simulink model "AutonomousDriving"  (R2018a)
settings: Solver=FixedStepAuto  StartTime=0.0  StopTime=inf  FixedStep=0.1  RelTol=1e-3
PreLoadFcn:
  | load('init.mat')
undefined symbols (not defined in the file): DiscIntNeverNeededParam, gray, init, Rec, SDTV
libraries: vrlib x7, simulink x3, PiCar_library x2, visionconversions x1
settings Model: Creator=al.hermann  LastModifiedBy=Tim

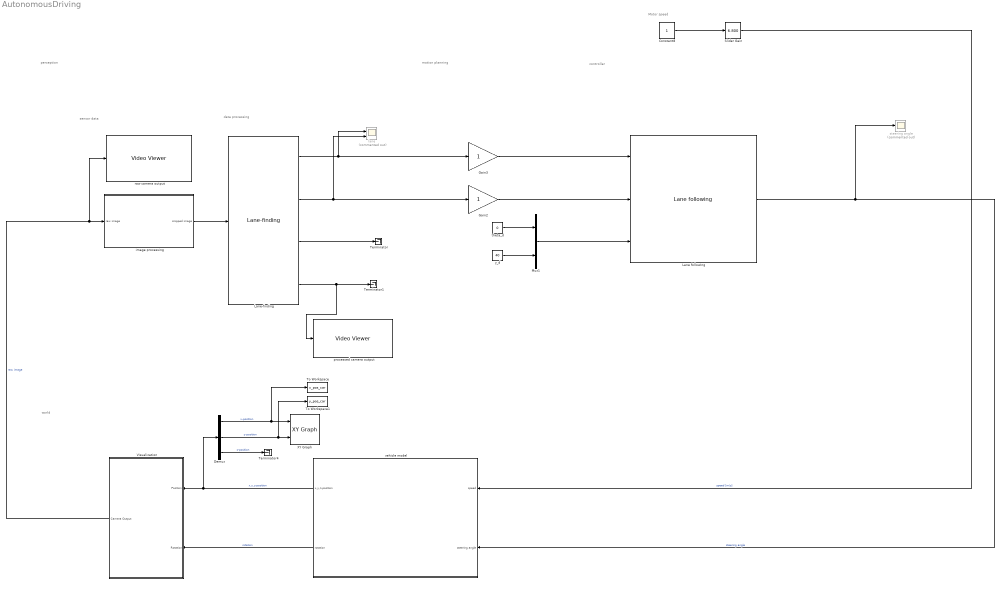
== system AutonomousDriving ==
  note: world
  note: motion planning
  note: controller
  note: perception
  note: data processing
  note: sensor data
  note: Motor speed
  Constant8 : Constant
  Demux : Demux  Outputs=3
  Gain2 : Gain
  Gain3 : Gain
  Lane following : PiCar_library/Lane following
      link override Discrete PID Controller: P=5  I=0  D=0
      link override K1: Gain=0
      link override Normalization: Gain=-1/300
  Lane-finding : PiCar_library/Lane-finding
  Mux1 : Mux  Inputs=2
  Slider Gain : simulink/Math Operations/Slider Gain  gain=6.800  low=0  high=10
  Terminator : Terminator
  Terminator1 : Terminator
  Terminator4 : Terminator
  To Workspace : ToWorkspace  VariableName=x_pos_car  SaveFormat=Timeseries  SampleTime=-1
  To Workspace1 : ToWorkspace  VariableName=y_pos_car  SaveFormat=Timeseries  SampleTime=-1
  Visualization : Subsystem
  XY Graph : simulink/Sinks/XY Graph  xmin=-400  xmax=500  ymin=-400  ymax=300  st=-1
  image processing : Subsystem
  lane : Scope  Commented=on  NumInputPorts=2
  processed camera output : VideoViewer  colormapValue=gray(256)  FigPos=[195 623 851 462]
  raw camera output : VideoViewer  colormapValue=gray(256)  FigPos=[632.428571428571 708.285714285714 737.714285714286 517.142857142857]
  steering angle : Scope  Commented=on
  theta_d : Constant  Value=0
  vehicle model : Subsystem
  y_d : Constant  Value=40
  wires:
  Visualization/1(Camera Output) -> raw camera output/1, image processing/1(raw image)  "raw image"
  Gain3/1 -> Lane following/1
  Mux1/1 -> Lane following/3
  theta_d/1 -> Mux1/1
  Gain2/1 -> Lane following/2
  y_d/1 -> Mux1/2
  Lane-finding/1 -> lane/1, Gain3/1
  Lane-finding/2 -> Gain2/1, lane/2
  Lane-finding/4 -> processed camera output/1, Terminator1/1
  Lane-finding/3 -> Terminator/1
  Slider Gain/1 -> vehicle model/1(speed)  "speed [m/s]"
  vehicle model/1(x,y,z-position) -> Demux/1, Visualization/1(Position)  "x,y,z-position"
  Lane following/1 -> vehicle model/2(steering angle), steering angle/1  "steering angle"
  vehicle model/2(rotation) -> Visualization/2(Rotation)  "rotation"
  image processing/1(cropped image) -> Lane-finding/1
  Demux/1 -> To Workspace/1, XY Graph/1  "x-position"
  Demux/2 -> To Workspace1/1, XY Graph/2  "y-position"
  Demux/3 -> Terminator4/1  "z-position"
  Constant8/1 -> Slider Gain/1

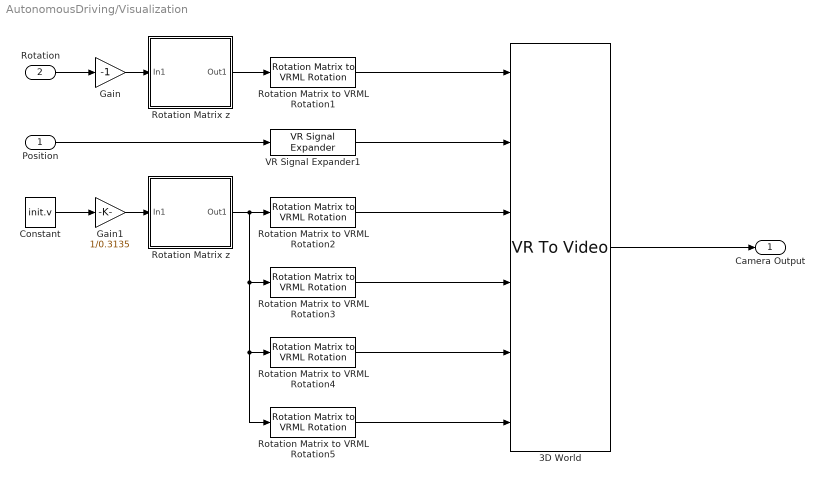
== system AutonomousDriving/Visualization ==
  Position : Inport
  Rotation : Inport  Port=2
  3D World : vrlib/VR To Video  InstantiateOnLoad=on  SampleTime=0.1  ViewEnable=on  RemoteChange=off  RemoteView=off  FieldsWritten=Car.rotation.4.1.1.double#Car.translation.3.1.1.double#RR_Rot.rotation.4.1.1.double#RL_Rot.rotation.4.1.1.double#FL_Rot.rotation.4.1.1.double#FR_Rot.rotation.4.1.1.double  WorldFileName=3DWorld.x3d  AutoView=off  VideoDimensions=[240 320]  AllowVariableSize=off  FigureProperties="{'Position', 'Name', 'Viewpoint', 'CameraBound', 'CameraDirection', 'CameraPosition', 'CameraUpVector', 'ZoomFactor', 'Antialiasing', 'Headlight', 'Lighting', 'NavPanel', 'Sound', 'StatusBar', 'Stereo3D', 'Stereo3DCameraOffset', 'Stereo3DHIT', 'ToolBar', 'Textures', 'Transparency', 'Triad', 'Wireframe', 'NavZones', 'NavMode', 'NavSpeed', 'CaptureFileFormat', 'CaptureFileName', 'Record2DCompressMethod', 'Record2DCompressQuality', 'Record2D', 'Record2DFileName', 'Record2DFPS'; [3.0000000000000000e+01   6.0000000000000000e+01   3.2000000000000000e+02   2.4000000000000000e+02], '', 'CAR', 'on', [0.0000000000000000e+00   0.0000000000000000e+00  -1.0000000000000000e+00], [0.0000000000000000e+00   0.0000000000000000e+00   0.0000000000000000e+00], [0.0000000000000000e+00   1.0000000000000000e+00   0.0000000000000000e+00], [1.0000000000000000e+00], 'off', 'on', 'on', 'none', 'on', 'off', 'off', [1.0000000149011612e-01], [0.0000000000000000e+00], 'off', 'on', 'on', 'none', 'off', 'off', 'examine', 'normal', 'tif', '%f_anim_%n.tif', 'auto', [7.5000000000000000e+01], 'off', '***video***', 'auto'}"
      settings: SourceProductName=Simulink 3D Animation  SourceProductBaseCode=VR
  Constant : Constant  Value=init.v
  Gain : Gain  Gain=-1
  Gain1 : Gain  Gain=1/0.3135
  Rotation Matrix to VRML Rotation{1..5} (5 alike) : vrlib/Utilities/Rotation Matrix to VRML Rotation  maxzero=1e-12
      settings: SourceProductName=Simulink 3D Animation  SourceProductBaseCode=VR
  Rotation Matrix z : Subsystem
  "Rotation Matrix z " : Subsystem
  VR Signal Expander1 : vrlib/VR Signal Expander  outwidth=3  outidx=[1 2 3]
      settings: SourceProductName=Simulink 3D Animation  SourceProductBaseCode=VR
  Camera Output : Outport
  wires:
  Rotation/1 -> Gain/1
  3D World/1 -> Camera Output/1
  Gain/1 -> Rotation Matrix z/1(In1)
  Position/1 -> VR Signal Expander1/1
  Rotation Matrix z/1(Out1) -> Rotation Matrix to VRML Rotation1/1
  Rotation Matrix to VRML Rotation1/1 -> 3D World/1
  VR Signal Expander1/1 -> 3D World/2
  Constant/1 -> Gain1/1
  Gain1/1 -> "Rotation Matrix z "/1(In1)
  "Rotation Matrix z "/1(Out1) -> Rotation Matrix to VRML Rotation3/1, Rotation Matrix to VRML Rotation5/1, Rotation Matrix to VRML Rotation4/1, Rotation Matrix to VRML Rotation2/1
  Rotation Matrix to VRML Rotation2/1 -> 3D World/3
  Rotation Matrix to VRML Rotation3/1 -> 3D World/4
  Rotation Matrix to VRML Rotation4/1 -> 3D World/5
  Rotation Matrix to VRML Rotation5/1 -> 3D World/6

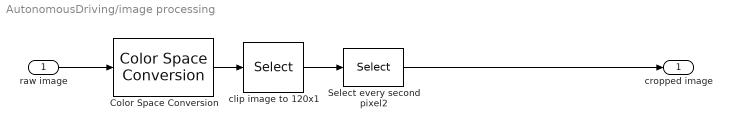
== system AutonomousDriving/image processing ==
  raw image : Inport
  Color Space Conversion : visionconversions/Color Space  Conversion  conversion=Obsolete  conversionActive=R'G'B' to intensity  wp_str=D65  rec=Rec. 601 (SDTV)  sys=1125/60/2:1  imagePorts=One multidimensional signal
      settings: SourceProductName=Computer Vision System Toolbox
  Select every second pixel2 : Selector  NumberOfDimensions=2  InputPortWidth=3  IndexOptions=Select all,Index vector (dialog)  Indices=[1:2:80],[1:2:160]  OutputSizes=1,1
  clip image to 120x1 : Selector  NumberOfDimensions=2  InputPortWidth=3  IndexOptions=Index vector (dialog),Index vector (dialog)  Indices=[120:1:194],[1:2:320]  OutputSizes=320,120
  cropped image : Outport
  wires:
  Select every second pixel2/1 -> cropped image/1
  Color Space Conversion/1 -> clip image to 120x1/1
  clip image to 120x1/1 -> Select every second pixel2/1
  raw image/1 -> Color Space Conversion/1

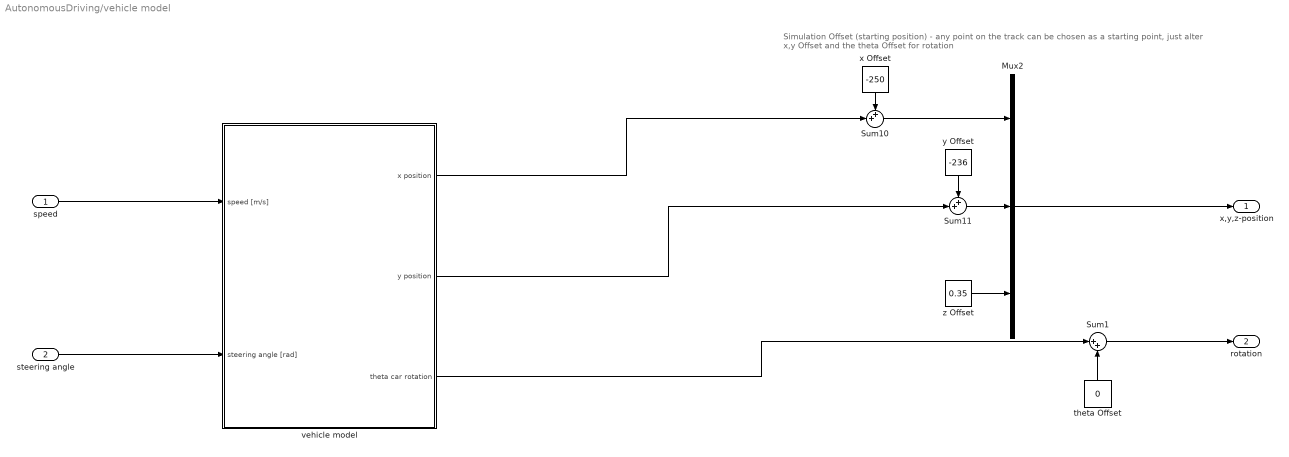
== system AutonomousDriving/vehicle model ==
  note: Simulation Offset (starting position) - any point on the track can be chosen
      | as a starting point, just alter x,y Offset and the theta Offset for rotation
  speed : Inport
  steering angle : Inport  Port=2
  Mux2 : Mux  Inputs=3
  Sum1 : Sum  Inputs=|++
  Sum10 : Sum  Inputs=++|
  Sum11 : Sum  Inputs=++|
  theta Offset : Constant  Value=0
  "vehicle model " : Subsystem
  x Offset : Constant  Value=-250
  y Offset : Constant  Value=-236
  z Offset : Constant  Value=0.35
  x,y,z-position : Outport
  rotation : Outport  Port=2
  wires:
  Mux2/1 -> x,y,z-position/1
  y Offset/1 -> Sum11/1
  z Offset/1 -> Mux2/3
  Sum10/1 -> Mux2/1
  x Offset/1 -> Sum10/1
  Sum11/1 -> Mux2/2
  Sum1/1 -> rotation/1
  theta Offset/1 -> Sum1/2
  speed/1 -> "vehicle model "/1(speed [m/s])
  steering angle/1 -> "vehicle model "/2(steering angle [rad])
  "vehicle model "/1(x position) -> Sum10/2
  "vehicle model "/2("y position ") -> Sum11/2
  "vehicle model "/3(theta car rotation) -> Sum1/1

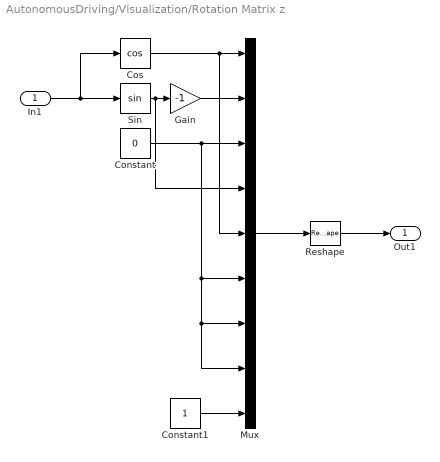
== system AutonomousDriving/Visualization/Rotation Matrix z ==
  In1 : Inport
  Constant : Constant  Value=0
  Constant1 : Constant
  Cos : Trigonometry  Operator=cos
  Gain : Gain  Gain=-1
  Mux : Mux  Inputs=9
  Reshape : Reshape  OutputDimensionality=Customize  OutputDimensions=[3, 3]
  Sin : Trigonometry
  Out1 : Outport
  wires:
  Reshape/1 -> Out1/1
  In1/1 -> Sin/1, Cos/1
  Mux/1 -> Reshape/1
  Cos/1 -> Mux/5, Mux/1
  Sin/1 -> Mux/4, Gain/1
  Constant/1 -> Mux/3, Mux/6, Mux/7, Mux/8
  Gain/1 -> Mux/2
  Constant1/1 -> Mux/9

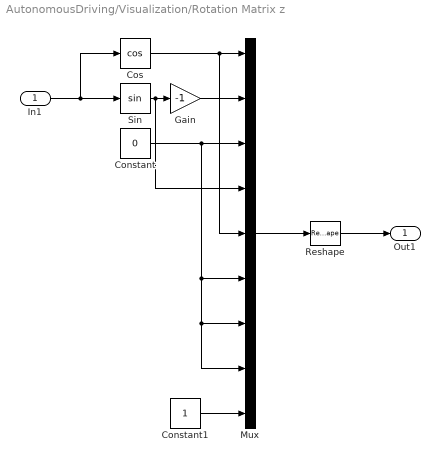
== system AutonomousDriving/Visualization/Rotation Matrix z  ==
  In1 : Inport
  Constant : Constant  Value=0
  Constant1 : Constant
  Cos : Trigonometry  Operator=cos
  Gain : Gain  Gain=-1
  Mux : Mux  Inputs=9
  Reshape : Reshape  OutputDimensionality=Customize  OutputDimensions=[3, 3]
  Sin : Trigonometry
  Out1 : Outport
  wires:
  Constant1/1 -> Mux/9
  Gain/1 -> Mux/2
  Constant/1 -> Mux/8, Mux/7, Mux/6, Mux/3
  Sin/1 -> Gain/1, Mux/4
  Cos/1 -> Mux/1, Mux/5
  Mux/1 -> Reshape/1
  In1/1 -> Cos/1, Sin/1
  Reshape/1 -> Out1/1

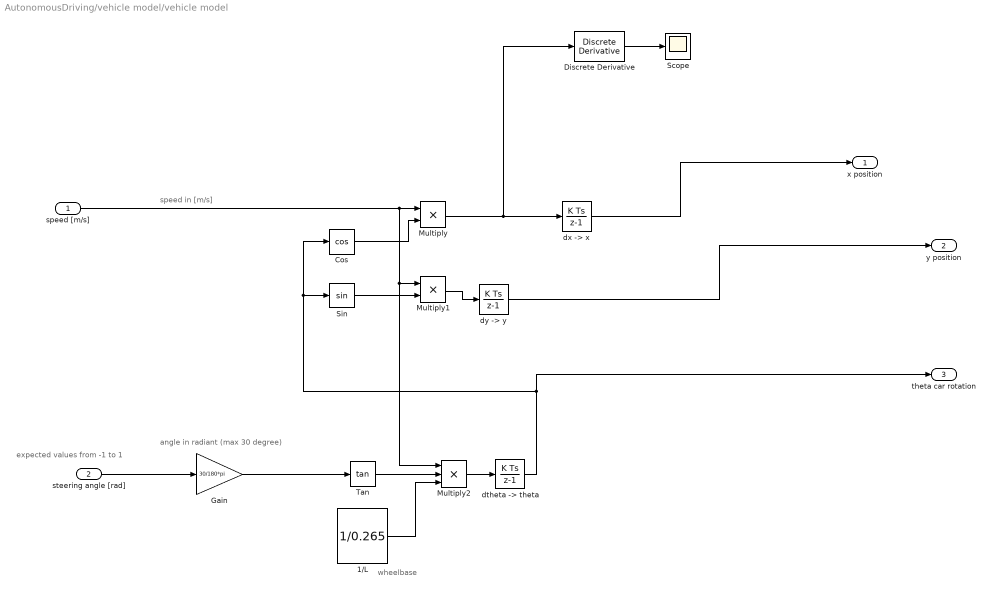
== system AutonomousDriving/vehicle model/vehicle model  ==
  note: angle in radiant (max 30 degree)
  note: expected values from -1 to 1
  note: wheelbase
  note: speed in [m/s]
  speed [m/s] : Inport
  steering angle [rad] : Inport  Port=2
  1/L : Constant  Value=1/0.265
  Cos : Trigonometry  Operator=cos
  Discrete Derivative : simulink/Discrete/Discrete Derivative  gainval=1.0  ICPrevScaledInput=0.0  OutMin=[]  OutMax=[]  OutDataType=fixdt(1, 16)  OutScaling=2^-10  DoSatur=off
  Gain : Gain  Gain=30/180*pi
  Multiply : Product
  Multiply1 : Product
  Multiply2 : Product  Inputs=3
  Scope : Scope
  Sin : Trigonometry
  Tan : Trigonometry  Operator=tan
  "dtheta -> theta" : DiscreteIntegrator  SampleTime=-1  ICPrevOutput=DiscIntNeverNeededParam  ICPrevScaledInput=DiscIntNeverNeededParam
  "dx -> x" : DiscreteIntegrator  SampleTime=-1  ICPrevOutput=DiscIntNeverNeededParam  ICPrevScaledInput=DiscIntNeverNeededParam
  "dy -> y" : DiscreteIntegrator  SampleTime=-1  ICPrevOutput=DiscIntNeverNeededParam  ICPrevScaledInput=DiscIntNeverNeededParam
  x position : Outport
  "y position " : Outport  Port=2
  theta car rotation : Outport  Port=3
  wires:
  Multiply2/1 -> "dtheta -> theta"/1
  Multiply/1 -> Discrete Derivative/1, "dx -> x"/1
  "dtheta -> theta"/1 -> theta car rotation/1, Sin/1, Cos/1
  Gain/1 -> Tan/1
  1/L/1 -> Multiply2/3
  speed [m/s]/1 -> Multiply2/1, Multiply1/1, Multiply/1
  Tan/1 -> Multiply2/2
  Sin/1 -> Multiply1/2
  Cos/1 -> Multiply/2
  Multiply1/1 -> "dy -> y"/1
  "dy -> y"/1 -> "y position "/1
  "dx -> x"/1 -> x position/1
  steering angle [rad]/1 -> Gain/1
  Discrete Derivative/1 -> Scope/1
